simulink model "just_model"  (R2019b)
settings: Solver=VariableStepAuto  StartTime=0.0  StopTime=15  RelTol=1e-3
values from neighbouring files (symbols this model uses):
  C_T = 0.0000363    (= 3.63e-05)    [calculate_w_from_f_m.m]    (also in create_model-mummel-PC.m; create_model.m)
  D_l = -diag([X_u_u Y_v_v Z_w_w K_p_p M_q_q N_r_r])    [create_model-mummel-PC.m]    (also in create_model.m)
  D_r = -diag([X_u_u Y_v_v Z_w_w K_p_p M_q_q N_r_r])    [create_model-mummel-PC.m]    (also in create_model.m)
  F_to_xrpy = [1 1 1 1;k_m -k_m k_m -k_m ; -h/2 -h/2 h/2 h/2 ; h/2 -h/2 -h/2 h/2]    [calculate_w_from_f_m.m]    (also in create_model-mummel-PC.m = [1 1 1 1;-k_m k_m -k_m k_m ; -h/2 -h/2 h/2 h/2 ; h/2 -h/2 -h; create_model.m = [1 1 1 1;-k_m k_m -k_m k_m ; -h/2 -h/2 h/2 h/2 ; h/2 -h/2 -h)
  m = 1.47    [create_model-mummel-PC.m]    (also in create_model.m)
  M_A_11 = M_A(1:3,1:3)    [create_model-mummel-PC.m]    (also in create_model.m)
  M_A_22 = M_A(4:6,4:6)    [create_model-mummel-PC.m]    (also in create_model.m)
  M_RB_22 = M_RB(4:6,4:6)    [create_model-mummel-PC.m]    (also in create_model.m)
  M_RB_M_A_INV = inv(M_RB+M_A)    [create_model-mummel-PC.m]    (also in create_model.m)
  mix_matrix_trpy_to_velocity_motor = [[1 1 1 1]' [-1 1 -1 1]' [-1 -1 1 1]' [1 -1 -1 1]']*0.4    [check_correct_index.m]    (also in create_model-mummel-PC.m = [[1 1 1 1]' [-1 1 -1 1]' [-1 -1 1 1]' [1 -1 -1 1]']; create_model.m = [[1 1 1 1]' [-1 1 -1 1]' [-1 -1 1 1]' [1 -1 -1 1]'])
settings Model: Creator=mummel  LastModifiedBy=mummel

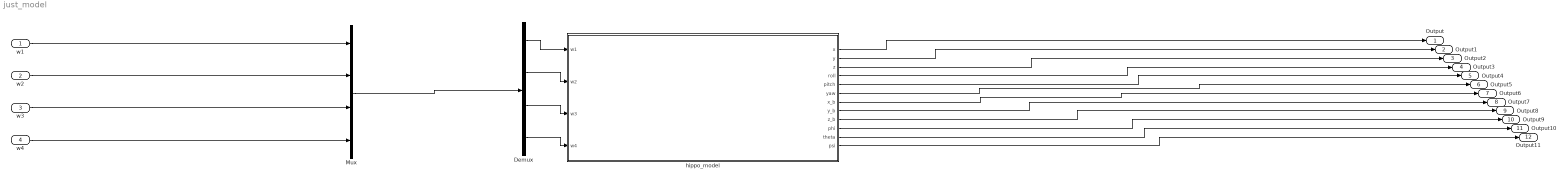
== system just_model ==
  w1 : Inport
  w2 : Inport  Port=2
  w3 : Inport  Port=3
  w4 : Inport  Port=4
  Demux : Demux
  Mux : Mux
  hippo_model : Subsystem
  Output : Outport
  Output1 : Outport  Port=2
  Output2 : Outport  Port=3
  Output3 : Outport  Port=4
  Output4 : Outport  Port=5
  Output5 : Outport  Port=6
  Output6 : Outport  Port=7
  Output7 : Outport  Port=8
  Output8 : Outport  Port=9
  Output9 : Outport  Port=10
  Output10 : Outport  Port=11
  Output11 : Outport  Port=12
  wires:
  w4/1 -> Mux/4
  w3/1 -> Mux/3
  w2/1 -> Mux/2
  w1/1 -> Mux/1
  hippo_model/1(x) -> Output/1
  hippo_model/2(y) -> Output1/1
  hippo_model/3(z) -> Output2/1
  hippo_model/4(roll) -> Output3/1
  hippo_model/5(pitch) -> Output4/1
  hippo_model/6(yaw) -> Output5/1
  hippo_model/7(x_b) -> Output6/1
  hippo_model/8(y_b) -> Output7/1
  hippo_model/9(z_b) -> Output8/1
  hippo_model/10(phi) -> Output9/1
  hippo_model/11(theta) -> Output10/1
  hippo_model/12(psi) -> Output11/1
  Mux/1 -> Demux/1
  Demux/1 -> hippo_model/1(w1)
  Demux/2 -> hippo_model/2(w2)
  Demux/3 -> hippo_model/3(w3)
  Demux/4 -> hippo_model/4(w4)

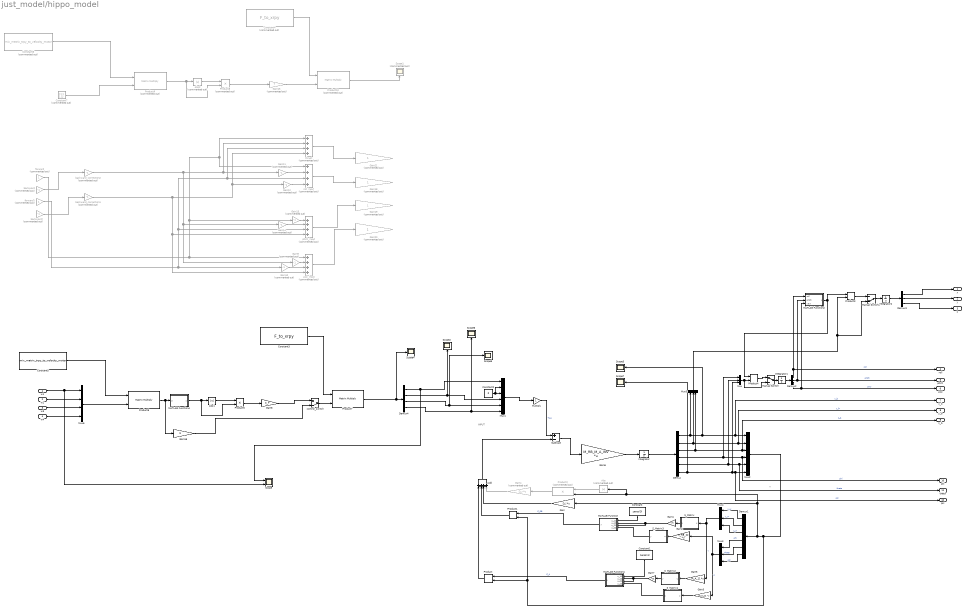
== system just_model/hippo_model ==
  note: INPUT
  note: v
  w1 : Inport
  w2 : Inport  Port=2
  w3 : Inport  Port=3
  w4 : Inport  Port=4
  Abs : Abs  Commented=on
  Abs1 : Abs
  Abs2 : Abs  Commented=on
  Add : Sum  Inputs=++++
  Constant : Constant  Value=zeros(3)
  Constant1 : Constant  Value=zeros(3)
  Constant2 : Constant  Value=0
  Constant3 : Constant  Value=F_to_xrpy
  Constant4 : Constant  Commented=on  Value=F_to_xrpy
  Constant5 : Constant  Value=mix_matrix_trpy_to_velocity_motor
  Constant6 : Constant  Commented=on  Value=mix_matrix_trpy_to_velocity_motor
  Constant7 : Constant  Commented=on  Value=[1 1 1 1]'
  Demux : Demux  Outputs=6
  Demux1 : Demux  Outputs=6
  Demux2 : Demux  Outputs=3
  Demux3 : Demux  Outputs=3
  Demux4 : Demux
  Gain : Gain  Gain=D_l  Multiplication=Matrix(K*u)
  Gain1 : Gain  Gain=-m
  Gain{9..14} (6 alike) : Gain  Commented=on  Gain=-1
  Gain15 : Gain  Commented=on  Gain=7
  Gain16 : Gain  Gain=9
  Gain{18..21} (4 alike) : Gain  Commented=on
  Gain2 : Gain  Gain=M_RB_22  Multiplication=Matrix(K*u)
  Gain3 : Gain  Gain=M_A_22  Multiplication=Matrix(K*u)
  Gain4 : Gain  Commented=on  Gain=D_r  Multiplication=Matrix(K*u)
  Gain5 : Gain  Gain=M_A_11  Multiplication=Matrix(K*u)
  Gain6 : Gain  Gain=M_RB_M_A_INV  Multiplication=Matrix(K*u)
  Gain7 : Gain  Gain=-m
  Gain8 : Gain  Gain=C_T
  Integrator : Integrator  ContinuousStateAttributes={'x_b', 'y_b', 'z_b','phi', 'theta', 'psi'}
  Integrator1 : Integrator  InitialCondition=[0 0 0]  ContinuousStateAttributes={'roll', 'pitch', 'yaw'}
  Integrator2 : Integrator  ContinuousStateAttributes={'x', 'y', 'z'}
  MATLAB Function : MATLAB Function  TreatAsAtomicUnit=on
  MATLAB Function1 : MATLAB Function  TreatAsAtomicUnit=on
  MATLAB Function2 : MATLAB Function  TreatAsAtomicUnit=on
  MATLAB Function4 : MATLAB Function  TreatAsAtomicUnit=on
  Manual Switch : ManualSwitch
  Manual Switch1 : ManualSwitch  CurrentSetting=0
  Multiply : Gain
  Mux{,3..5} (4 alike) : Mux  Inputs=3
  Mux1 : Mux  Inputs=6
  Mux2 : Mux  Inputs=6
  Mux6 : Mux
  Product{,1,3..4,6..7} (6 alike) : Product  Multiplication=Matrix(*)
  Product10 : Product  Commented=on  Multiplication=Matrix(*)
  Product2 : Product  Commented=on
  Product5 : Product
  Product8 : Product  Commented=on
  Product9 : Product  Commented=on  Multiplication=Matrix(*)
  S_Matrix : MATLAB Function  TreatAsAtomicUnit=on
  S_Matrix1 : MATLAB Function  TreatAsAtomicUnit=on
  S_Matrix2 : MATLAB Function  TreatAsAtomicUnit=on
  S_Matrix3 : MATLAB Function  TreatAsAtomicUnit=on
  Scope : Scope  NumInputPorts=2
  Scope1 : Scope  Commented=on
  Scope{2..7} (6 alike) : Scope
  Subtract : Sum  Inputs=+-
  backward : Gain  Commented=on  Gain=-1
  backward1 : Gain  Commented=on  Gain=-1
  backward_correction1 : Gain  Commented=on  Gain=-1
  backward_correction2 : Gain  Commented=on  Gain=-1
  control_switch : ManualSwitch  CurrentSetting=0
  forward : Gain  Commented=on
  forward1 : Gain  Commented=on
  pitch_input : Sum  Commented=on  Inputs=++++
  roll_input : Sum  Commented=on  Inputs=++++
  thrust : Sum  Commented=on  Inputs=++++
  yaw_input : Sum  Commented=on  Inputs=++++
  x : Outport
  y : Outport  Port=2
  z : Outport  Port=3
  roll : Outport  Port=4
  pitch : Outport  Port=5
  yaw : Outport  Port=6
  x_b : Outport  Port=7
  y_b : Outport  Port=8
  z_b : Outport  Port=9
  phi : Outport  Port=10
  theta : Outport  Port=11
  psi : Outport  Port=12
  wires:
  Demux/6 -> Scope7/1, Mux/3, psi/1, Mux2/6  "psi"
  S_Matrix3/1(y) -> MATLAB Function/4(u_22)
  Demux/5 -> Mux/2, theta/1, Mux2/5  "theta"
  Gain1/1 -> MATLAB Function/3(u_21), MATLAB Function/2(u_12)
  Mux1/1 -> Multiply/1
  Gain6/1 -> Integrator/1
  MATLAB Function1/1(y) -> Product/1  "C_A"
  Demux2/3 -> yaw/1, MATLAB Function2/3(yaw)  "yaw"
  Demux/2 -> y_b/1, Mux2/2, Mux5/2  "y_b"
  Demux2/2 -> pitch/1, MATLAB Function2/2(pitch)  "pitch"
  Demux/4 -> Mux/1, phi/1, Mux2/4  "phi"
  Integrator1/1 -> Demux2/1
  MATLAB Function/1(y) -> Product1/1  "C_RB"
  S_Matrix/1(y) -> Gain1/1
  Product1/1 -> Add/2
  Constant1/1 -> MATLAB Function1/1(u_11)
  Gain7/1 -> MATLAB Function1/2(u_12), MATLAB Function1/3(u_21)
  Gain/1 -> Add/3
  Demux2/1 -> MATLAB Function2/1(roll), roll/1  "roll"
  Demux/3 -> z_b/1, Mux2/3, Mux5/3  "z_b"
  Add/1 -> Subtract/2
  Product/1 -> Add/1
  Demux/1 -> Scope3/1, x_b/1, Mux2/1, Mux5/1  "x_b"
  Mux2/1 -> Product/2, Product1/2, Abs/1, Product2/2, Gain/1, Demux1/1
  Constant2/1 -> Mux1/2, Mux1/3
  Product2/1 -> Gain4/1
  Demux1/5 -> Mux3/2  "theta"
  Mux3/1 -> Gain3/1, Gain2/1  "w"
  Gain4/1 -> Add/4
  S_Matrix1/1(y) -> MATLAB Function1/4(u_22)
  Gain3/1 -> S_Matrix1/1(u)
  Integrator/1 -> Demux/1
  Multiply/1 -> Subtract/1  "TAU"
  S_Matrix2/1(y) -> Gain7/1
  Demux1/3 -> Mux4/3  "z_w"
  Demux1/4 -> Mux3/1  "phi"
  Demux1/6 -> Mux3/3  "psi"
  Subtract/1 -> Gain6/1
  Product3/1 -> Manual Switch1/1
  Mux4/1 -> S_Matrix/1(u), Gain5/1  "v"
  Abs/1 -> Product2/1
  Gain2/1 -> S_Matrix3/1(u)
  Mux5/1 -> Product3/2, Manual Switch1/2
  MATLAB Function2/1(y) -> Product3/1, Product4/1
  Gain5/1 -> S_Matrix2/1(u)
  Demux3/2 -> y/1
  Demux1/1 -> Mux4/1  "x_w"
  Constant/1 -> MATLAB Function/1(u_11)
  Demux1/2 -> Mux4/2  "y_w"
  Demux3/1 -> x/1
  Demux3/3 -> z/1
  thrust/1 -> Gain21/1
  forward/1 -> roll_input/1, thrust/1, Gain13/1, yaw_input/1
  backward/1 -> backward_correction2/1
  forward1/1 -> roll_input/3, thrust/3, pitch_input/3, Gain10/1
  backward1/1 -> backward_correction1/1
  backward_correction2/1 -> Gain9/1, Gain14/1, Gain11/1, thrust/2
  backward_correction1/1 -> thrust/4, Gain12/1, yaw_input/4, pitch_input/4
  roll_input/1 -> Gain18/1
  Gain9/1 -> yaw_input/2
  Gain10/1 -> yaw_input/3
  Gain12/1 -> roll_input/4
  Gain11/1 -> roll_input/2
  yaw_input/1 -> Gain20/1
  Gain14/1 -> pitch_input/2
  Gain13/1 -> pitch_input/1
  pitch_input/1 -> Gain19/1
  Integrator2/1 -> Demux3/1
  Manual Switch/1 -> Integrator1/1
  Mux/1 -> Manual Switch/2, Product4/2
  Product4/1 -> Manual Switch/1
  Manual Switch1/1 -> Integrator2/1
  Demux4/1 -> Scope/1, Mux1/1
  Demux4/2 -> Scope2/1, Mux1/4
  Demux4/4 -> Mux1/6, Scope6/1
  Demux4/3 -> Scope5/1, Mux1/5
  w1/1 -> Scope/2, Mux6/1
  w2/1 -> Mux6/2
  w3/1 -> Mux6/3
  w4/1 -> Mux6/4
  Constant3/1 -> Product7/1
  MATLAB Function4/1(y) -> Abs1/1, Product5/2
  Constant5/1 -> Product6/1
  Abs1/1 -> Product5/1
  Gain8/1 -> control_switch/1
  Mux6/1 -> Product6/2
  Product7/1 -> Scope4/1, Demux4/1
  Constant4/1 -> Product10/1
  Constant7/1 -> Product9/2
  Product8/1 -> Gain15/1
  Constant6/1 -> Product9/1
  Abs2/1 -> Product8/1
  Gain15/1 -> Product10/2
  Product9/1 -> Product8/2, Abs2/1
  Product10/1 -> Scope1/1
  Product5/1 -> Gain8/1
  Product6/1 -> Gain16/1, MATLAB Function4/1(p)
  Gain16/1 -> control_switch/2
  control_switch/1 -> Product7/2

== matlab function just_model/hippo_model/MATLAB Function1 ==
  data: u_11 input; y output; u_12 input; u_21 input; u_22 input
function y = fcn(u_11,u_12,u_21,u_22)

y = [u_11 u_12; u_21 u_22];

== matlab function just_model/hippo_model/MATLAB Function ==
  data: u_11 input; y output; u_12 input; u_21 input; u_22 input
function y = fcn(u_11,u_12,u_21,u_22)

y = [u_11 u_12; u_21 u_22];

== matlab function just_model/hippo_model/S_Matrix ==
  data: u input size=3; y output
function y = fcn(u)

y = cross(repmat(u,1,3),eye(3,3)) ;

== matlab function just_model/hippo_model/S_Matrix1 ==
  data: u input; y output
function y = fcn(u)

y = cross(repmat(u,1,3),eye(3,3)) ;

== matlab function just_model/hippo_model/S_Matrix2 ==
  data: u input; y output
function y = fcn(u)
y = cross(repmat(u,1,3),eye(3,3)) ;

== matlab function just_model/hippo_model/S_Matrix3 ==
  data: u input size=3; y output
function y = fcn(u)

y = cross(repmat(u,1,3),eye(3,3)) ;

== matlab function just_model/hippo_model/MATLAB Function2 ==
  data: roll input; y output; pitch input; yaw input
function y = fcn(roll,pitch,yaw)
alpha = yaw;
beta = pitch;
gamma = roll;
R_roll=[1 0 +sin(pitch);0 cos(roll) -sin(roll)+sin(pitch);0 sin(roll) cos(roll)];
%R_roll=[1 0 0;0 cos(roll) -sin(roll);0 sin(roll) cos(roll)]
% R_pitch=[cos(pitch) 0 sin(pitch);0 1 0; -sin(pitch) 0 cos(pitch)]
% R_yaw=[cos(yaw) -sin(yaw) 0; sin(yaw) cos(yaw) 0; 0 0 1]



%R=[cos(alpha)*cos(beta) cos(alpha)*sin(beta)*sin(gamma)-sin(alpha)*cos(gamma) cos(alpha)*sin(beta)*cos(gamma)+sin(alpha)*sin(gamma);
%  sin(alpha)*cos(beta) sin(alpha)*sin(beta)*sin(gamma)+cos(alpha)*cos(gamma) sin(alpha)*sin(beta)*cos(gamma)-cos(alpha)*sin(gamma);
%  -sin(beta) cos(beta)*sin(gamma) cos(beta)*cos(gamma)];
y = R_roll;

== matlab function just_model/hippo_model/MATLAB Function4 ==
  data: p input; y output
function y = fcn(p)

u=[0 0 0 0]';


u(1)=p(1);
u(2)=p(2);
u(3)=p(3);
u(4)=p(4);
for i=1:4
    if(u(i)>1)
        u(i)=1;
    end
    if(u(i)<-1)
        u(i)=-1;
    end
end

u=500*u;


%if max(abs(u))>500
%    u=u/max(abs(u))*500
%end
y = u;
